simulink model "modelV1_2"  (R2024b)
settings: Solver=VariableStepAuto  StartTime=0.0  StopTime=30  RelTol=1e-3
values from neighbouring files (symbols this model uses):
  prop =     [F15_thrust.mat]
undefined symbols (not defined in the file or in its folder): DiscIntNeverNeededParam
libraries: simulink x2, slpidlib x1
settings Model: Creator=C27Lucan.Keyser  LastModifiedBy=lucan

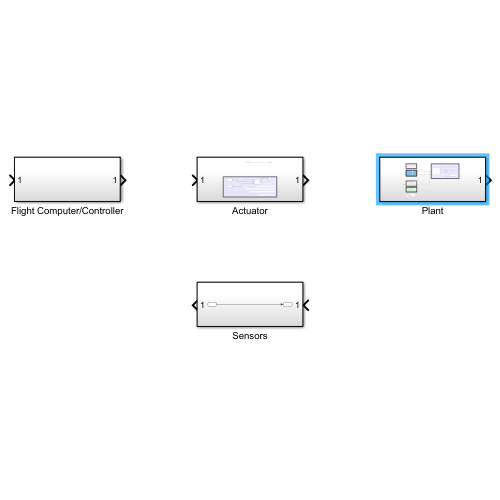
[thumbnail: Simulink's stored preview of the top-level diagram]
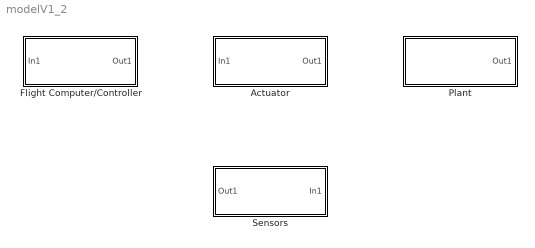
== system modelV1_2 ==
  Actuator : Subsystem
  Flight Computer/Controller : Subsystem
  Plant : Subsystem
  Sensors : Subsystem

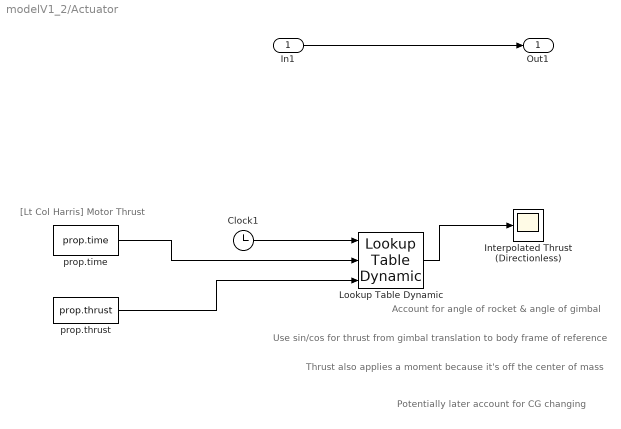
== system modelV1_2/Actuator ==
  note: Potentially later account for CG changing
  note: Thrust also applies a moment because it's off the center of mass
  note: Account for angle of rocket & angle of gimbal
  note: [Lt Col Harris] Motor Thrust
  note: Use sin/cos for thrust from gimbal translation to body frame of reference
  In1 : Inport
  Clock1 : Clock
  Interpolated Thrust (Directionless) : Scope
  Lookup Table Dynamic : simulink/Lookup Tables/Lookup Table Dynamic  LookUpMeth=Interpolation-Use End Values  OutDataType=fixdt('double')  OutScaling=2^-10  OutputDataTypeScalingMode=Specify via dialog  OutDataTypeStr=double  DoSatur=off
  prop.thrust : Constant  Value=prop.thrust
  prop.time : Constant  Value=prop.time
  Out1 : Outport
  wires:
  In1/1 -> Out1/1
  prop.time/1 -> Lookup Table Dynamic/2
  prop.thrust/1 -> Lookup Table Dynamic/3
  Lookup Table Dynamic/1 -> Interpolated Thrust (Directionless)/1
  Clock1/1 -> Lookup Table Dynamic/1

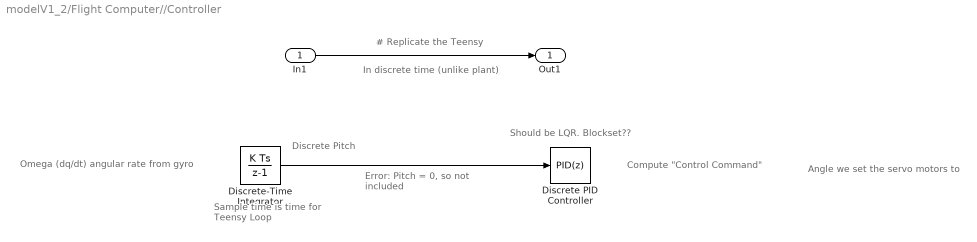
== system modelV1_2/Flight Computer//Controller ==
  note: Angle we set the servo motors to
  note: Error: Pitch = 0, so not included
  note: Should be LQR. Blockset??
  note: Discrete Pitch
  note: Sample time is time for Teensy Loop
  note: In discrete time (unlike plant)
  note: Omega (dq/dt) angular rate from gyro
  note: Compute "Control Command"
  note: # Replicate the Teensy
  In1 : Inport
  Discrete PID Controller : slpidlib/PID Controller  Controller=PID  Form=Parallel  TimeDomain=Discrete-time  UseExternalTs=off  SampleTime=-1  IntegratorMethod=Forward Euler  FilterMethod=Forward Euler  ControllerParametersSource=internal  P=1  I=1  UseKiTs=off  D=0  UseExternalDerivativeSource=off  N=100  UseFilter=on  TunerSelectOption=Transfer Function Based (PID Tuner App)  InitialConditionSource=internal  InitialConditionForIntegrator=0  InitialConditionForFilter=0  DifferentiatorICPrevScaledInput=0  ExternalReset=none  TrackingMode=off  Kt=1  LimitOutput=off  SatLimitsSource=internal  UpperSaturationLimit=inf  LowerSaturationLimit=-inf  LinearizeAsGain=off  AntiWindupMode=none  Kb=1  LimitIntegrator=off  UpperIntegratorSaturationLimit=inf  LowerIntegratorSaturationLimit=-inf  POutMin=[]  POutMax=[]  IOutMin=[]  IOutMax=[]  DOutMin=[]  DOutMax=[]  NOutMin=[]  NOutMax=[]  SumOutMin=[]  SumOutMax=[]  SaturationOutMin=[]  SaturationOutMax=[]  PParamMin=[]  PParamMax=[]  IParamMin=[]  IParamMax=[]  DParamMin=[]  DParamMax=[]  NParamMin=[]  NParamMax=[]  KbParamMin=[]  KbParamMax=[]  KtParamMin=[]  KtParamMax=[]  KbOutMin=[]  KbOutMax=[]  KtOutMin=[]  KtOutMax=[]  IntegratorOutMin=[]  IntegratorOutMax=[]  FilterOutMin=[]  FilterOutMax=[]  SumI1OutMin=[]  SumI1OutMax=[]  SumI2OutMin=[]  SumI2OutMax=[]  SumI3OutMin=[]  SumI3OutMax=[]  SumI4OutMin=[]  SumI4OutMax=[]  SumDOutMin=[]  SumDOutMax=[]  DifferentiatorOutMin=[]  DifferentiatorOutMax=[]  FilterDiffOutCoefMin=[]  FilterDiffOutCoefMax=[]  ReciprocalOutMin=[]  ReciprocalOutMax=[]  SumDenOutMin=[]  SumDenOutMax=[]  SumNumOutMin=[]  SumNumOutMax=[]  DivideOutMin=[]  DivideOutMax=[]  UdiffTsProdOutMin=[]  UdiffTsProdOutMax=[]  NTsProdOutMin=[]  NTsProdOutMax=[]  UintegralTsProdOutMin=[]  UintegralTsProdOutMax=[]  UngainTsProdOutMin=[]  UngainTsProdOutMax=[]  ClampingZeroOutDataTypeStr=Inherit: Inherit via back propagation  ClampingZeroOutMin=[]  ClampingZeroOutMax=[]  FilterDenConstantOutDataTypeStr=Inherit: Inherit via back propagation  FilterDenConstantOutMin=[]  FilterDenConstantOutMax=[]  PCopyOutDataTypeStr=Inherit: Inherit via back propagation  PCopyOutMin=[]  PCopyOutMax=[]  NCopyOutDataTypeStr=Inherit: Inherit via back propagation  NCopyOutMin=[]  NCopyOutMax=[]  IntegratorContinuousStateAttributes=''  IntegratorStateMustResolveToSignalObject=off  IntegratorRTWStateStorageClass=Auto  FilterContinuousStateAttributes=''  FilterStateMustResolveToSignalObject=off  FilterRTWStateStorageClass=Auto  ParallelPVariant=InternalParameters  IdealPVariant=Disabled  IVariant=InternalParameters  DVariant=InternalParameters  IntegratorVariant=Discrete  SatVariant=Disabled  AWVariant=Passthrough  PCopyVariant=Disabled  TRVariant=Disabled  FdbkBlocksVariant=Forward  IdealPFdbkVariant=Disabled  SatFdbkVariant=Disabled  DerivativeFilterVariant=ForwardEulerFilter  NVariant=InternalParameters  NCopyVariant=Disabled  FilterICVariant=InternalICsFilter  IntegratorICVariant=InternalICs  ExternalResetVariant=Disabled  TRSumVariant=Passthrough  SumFdbkVariant=Disabled  SumVariant=Sum_PID  TsampFilterVariant=InternalTs  TsampNgainVariant=Passthrough  TsampIntegralVariant=Passthrough  ExternalSaturationOutDataTypeStr=Inherit: Same as second input  DerivativeSourceVariant=ErrorSignal  PreIntVariant=InternalPreInt
      settings: LibrarySourceBlock=simulink/Discrete/Discrete PID Controller
  Discrete-Time Integrator : DiscreteIntegrator  SampleTime=0.01  ICPrevOutput=DiscIntNeverNeededParam  ICPrevScaledInput=DiscIntNeverNeededParam
  Out1 : Outport
  wires:
  In1/1 -> Out1/1
  ? -> Discrete-Time Integrator/1
  Discrete-Time Integrator/1 -> Discrete PID Controller/1

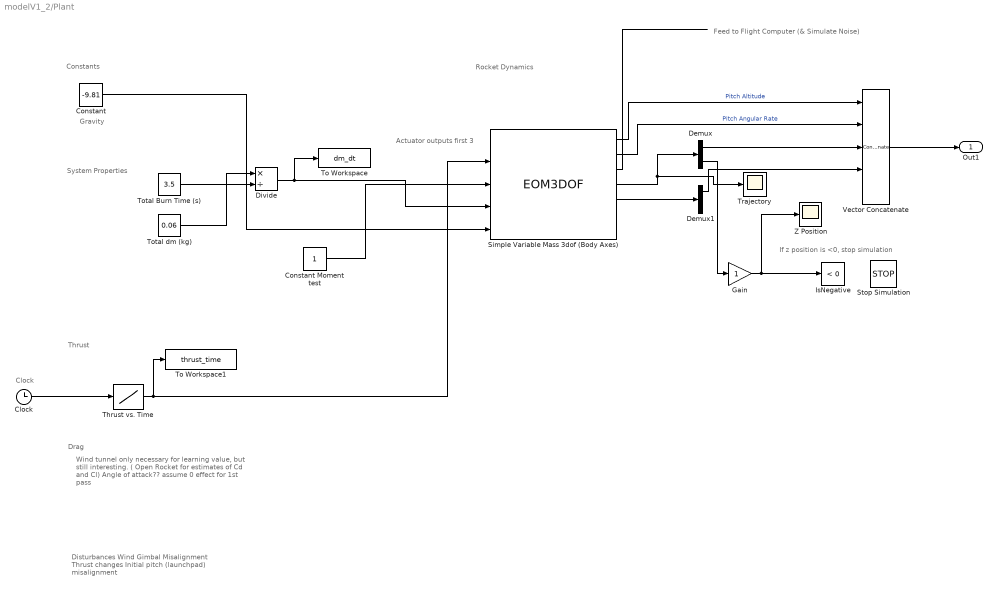
== system modelV1_2/Plant ==
  note: Disturbances
      | Wind
      | Gimbal Misalignment
      | Thrust changes
      | Initial pitch (launchpad) misalignment
  note: Feed to Flight Computer (& Simulate Noise)
  note: Wind tunnel only necessary for learning value, but still interesting. ( Open Rocket for estimates of Cd and Cl)
      |
      | Angle of attack?? assume 0 effect for 1st pass
  note: Actuator outputs first 3
  note: Gravity
  note: Clock
  note: System Properties
  note: If z position is <0, stop simulation
  note: Constants
  note: Rocket Dynamics
  note: Thrust
  note: Drag
  Clock : Clock
  Constant : Constant  Value=-9.81
  Constant Moment test : Constant
  Demux : Demux  Outputs=2
  Demux1 : Demux  Outputs=2
  Divide : Product  Inputs=*/  OutDataTypeStr=double
  Gain : Gain
  IsNegative : simulink/Logic and Bit Operations/Compare To Zero  relop=<  OutDataTypeStr=boolean
      settings: LibrarySourceBlock=|
      | simulink/Quick Insert/Logic and Bit
      | Operations/IsNegative
  Simple Variable Mass 3dof (Body Axes) : EOM3DOF  mtype=Simple Variable  mass_f=1.0  g_in=External
  Stop Simulation : Stop
  Thrust vs. Time : Lookup_n-D  NumberOfTableDimensions=1  BreakpointsForDimension1=prop.time  Table=prop.thrust  InternalRulePriority=Speed  RndMeth=Simplest
  To Workspace : ToWorkspace  VariableName=dm_dt  SampleTime=-1
  To Workspace1 : ToWorkspace  VariableName=thrust_time  SampleTime=-1
  Total Burn Time (s) : Constant  Value=3.5
  Total dm (kg) : Constant  Value=0.06
  Trajectory : Scope
  Vector Concatenate : Concatenate  NumInputs=5
  Z Position : Scope
  Out1 : Outport
  wires:
  Simple Variable Mass 3dof (Body Axes)/1 -> Vector Concatenate/1  "Pitch Altitude"
  Simple Variable Mass 3dof (Body Axes)/2 -> Vector Concatenate/2  "Pitch Angular Rate"
  Simple Variable Mass 3dof (Body Axes)/5 -> Demux1/1
  Simple Variable Mass 3dof (Body Axes)/4 -> Trajectory/1, Demux/1
  Demux/1 -> Vector Concatenate/3
  Demux1/1 -> Vector Concatenate/4
  Vector Concatenate/1 -> Out1/1
  Demux/2 -> Gain/1
  Gain/1 -> IsNegative/1, Z Position/1
  Constant/1 -> Simple Variable Mass 3dof (Body Axes)/5
  Divide/1 -> To Workspace/1, Simple Variable Mass 3dof (Body Axes)/4
  Total dm (kg)/1 -> Divide/1
  Total Burn Time (s)/1 -> Divide/2
  Clock/1 -> Thrust vs. Time/1
  Thrust vs. Time/1 -> To Workspace1/1, Simple Variable Mass 3dof (Body Axes)/2
  Constant Moment test/1 -> Simple Variable Mass 3dof (Body Axes)/3
  Simple Variable Mass 3dof (Body Axes)/3 -> ?

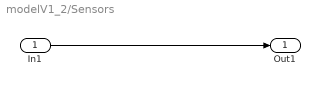
== system modelV1_2/Sensors ==
  In1 : Inport
  Out1 : Outport
  wires:
  In1/1 -> Out1/1
